simulink model "LHP_DT_v1"  (R2025b)
settings: Solver=VariableStepAuto  StartTime=0.0  StopTime=60  RelTol=1e-3
undefined symbols (not defined in the file): P
libraries: SignalEditorBlockLib x1
settings Model: Creator=RayAlmighty  LastModifiedBy=rayom

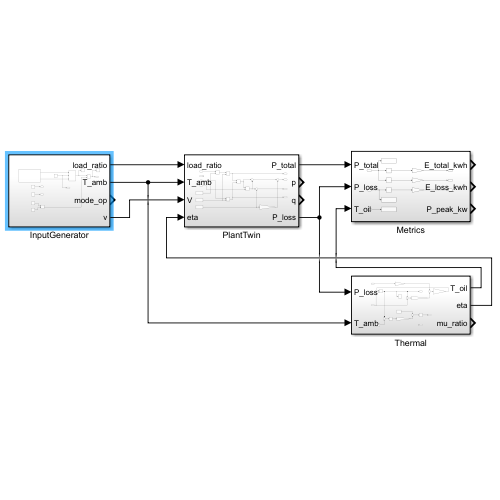
[thumbnail: Simulink's stored preview of the top-level diagram]
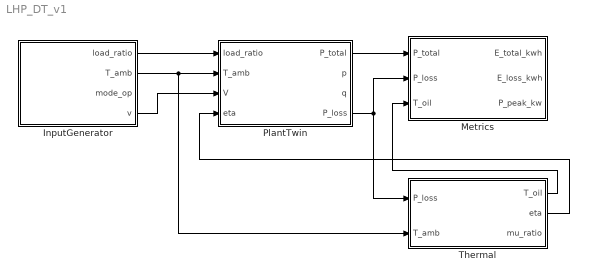
== system LHP_DT_v1 ==
  InputGenerator : Subsystem
  Metrics : Subsystem
  PlantTwin : Subsystem
  Thermal : Subsystem
  wires:
  InputGenerator/2(T_amb) -> Thermal/2(T_amb), PlantTwin/2(T_amb)
  InputGenerator/1(load_ratio) -> PlantTwin/1(load_ratio)
  InputGenerator/4(v) -> PlantTwin/3(V)
  Thermal/2(eta) -> PlantTwin/4(eta)
  PlantTwin/4(P_loss) -> Metrics/2(P_loss), Thermal/1(P_loss)
  PlantTwin/1(P_total) -> Metrics/1(P_total)
  Thermal/1(T_oil) -> Metrics/3(T_oil)

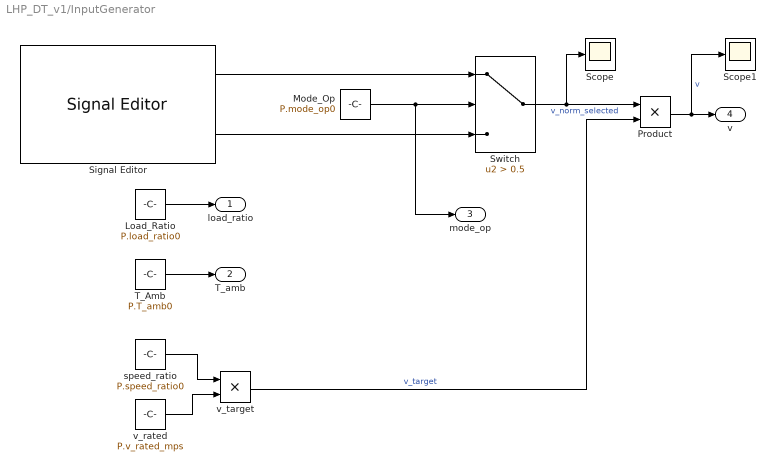
== system LHP_DT_v1/InputGenerator ==
  Load_Ratio : Constant  Value=P.load_ratio0
  Mode_Op : Constant  Value=P.mode_op0
  Product : Product
  Scope : Scope
      settings: ActiveDisplayYMinimum=-1  ActiveDisplayYMaximum=1
  Scope1 : Scope
      settings: ActiveDisplayYMinimum=-1  ActiveDisplayYMaximum=1  DataLoggingVariableName=ScopeData2
  Signal Editor : SignalEditorBlockLib/Signal Editor  FileName=v_norm.mat  ActiveScenario=Scenario  ActiveSignal=v_smooth  IsBus=off  OutputBusObjectStr=Bus: BusObject  SampleTime=0  ZeroCross=off  OutputAfterFinalValue=Setting to zero  Unit=inherit  PreserveSignalName=on  ApplySigPropsToAllScenarios=on  ApplySigPropsToAllSignals=off  SignalPropertySource=Dialog parameters
  Switch : Switch  Criteria=u2 > Threshold  Threshold=0.5  SaturateOnIntegerOverflow=off  InputSameDT=off
  T_Amb : Constant  Value=P.T_amb0
  speed_ratio : Constant  Value=P.speed_ratio0
  v_rated : Constant  Value=P.v_rated_mps
  v_target : Product
  load_ratio : Outport
  T_amb : Outport  Port=2
  mode_op : Outport  Port=3
  v : Outport  Port=4
  wires:
  Signal Editor/2 -> Switch/3
  Mode_Op/1 -> mode_op/1, Switch/2
  Switch/1 -> Product/1, Scope/1  "v_norm_selected"
  Load_Ratio/1 -> load_ratio/1
  T_Amb/1 -> T_amb/1
  speed_ratio/1 -> v_target/1
  v_rated/1 -> v_target/2
  v_target/1 -> Product/2  "v_target"
  Product/1 -> Scope1/1, v/1  "v"
  Signal Editor/1 -> Switch/1

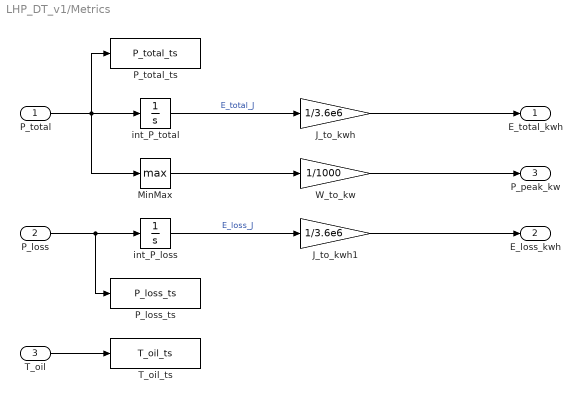
== system LHP_DT_v1/Metrics ==
  P_total : Inport
  P_loss : Inport  Port=2
  T_oil : Inport  Port=3
  J_to_kwh : Gain  Gain=1/3.6e6
  J_to_kwh1 : Gain  Gain=1/3.6e6
  MinMax : MinMax  Function=max
  P_loss_ts : ToWorkspace  VariableName=P_loss_ts  SaveFormat=Timeseries  SampleTime=-1
  P_total_ts : ToWorkspace  VariableName=P_total_ts  SaveFormat=Timeseries  SampleTime=-1
  T_oil_ts : ToWorkspace  VariableName=T_oil_ts  SaveFormat=Timeseries  SampleTime=-1
  W_to_kw : Gain  Gain=1/1000
  int_P_loss : Integrator
  int_P_total : Integrator
  E_total_kwh : Outport
  E_loss_kwh : Outport  Port=2
  P_peak_kw : Outport  Port=3
  wires:
  P_total/1 -> P_total_ts/1, int_P_total/1, MinMax/1
  int_P_total/1 -> J_to_kwh/1  "E_total_J"
  J_to_kwh/1 -> E_total_kwh/1
  P_loss/1 -> P_loss_ts/1, int_P_loss/1
  int_P_loss/1 -> J_to_kwh1/1  "E_loss_J"
  J_to_kwh1/1 -> E_loss_kwh/1
  MinMax/1 -> W_to_kw/1
  W_to_kw/1 -> P_peak_kw/1
  T_oil/1 -> T_oil_ts/1

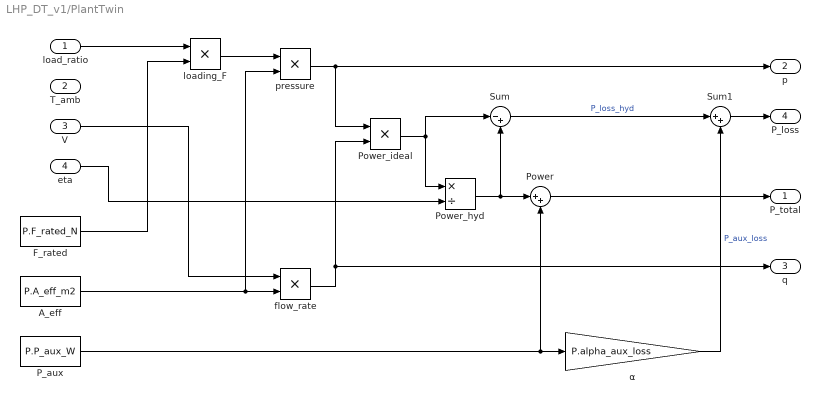
== system LHP_DT_v1/PlantTwin ==
  load_ratio : Inport
  T_amb : Inport  Port=2
  V : Inport  Port=3
  eta : Inport  Port=4
  A_eff : Constant  Value=P.A_eff_m2
  F_rated : Constant  Value=P.F_rated_N
  P_aux : Constant  Value=P.P_aux_W
  Power : Sum  Inputs=|++
  Power_hyd : Product  Inputs=*/
  Power_ideal : Product
  Sum : Sum  Inputs=|-+
  Sum1 : Sum  Inputs=|++
  flow_rate : Product
  loading_F : Product
  pressure : Product
  α : Gain  Gain=P.alpha_aux_loss
  P_total : Outport
  p : Outport  Port=2
  q : Outport  Port=3
  P_loss : Outport  Port=4
  wires:
  load_ratio/1 -> loading_F/1
  F_rated/1 -> loading_F/2
  loading_F/1 -> pressure/1
  A_eff/1 -> pressure/2, flow_rate/2
  V/1 -> flow_rate/1
  pressure/1 -> Power_ideal/1, p/1
  flow_rate/1 -> Power_ideal/2, q/1
  Power_ideal/1 -> Sum/1, Power_hyd/1
  P_aux/1 -> Power/2, α/1
  Power/1 -> P_total/1
  eta/1 -> Power_hyd/2
  Power_hyd/1 -> Sum/2, Power/1
  α/1 -> Sum1/2  "P_aux_loss"
  Sum/1 -> Sum1/1  "P_loss_hyd"
  Sum1/1 -> P_loss/1

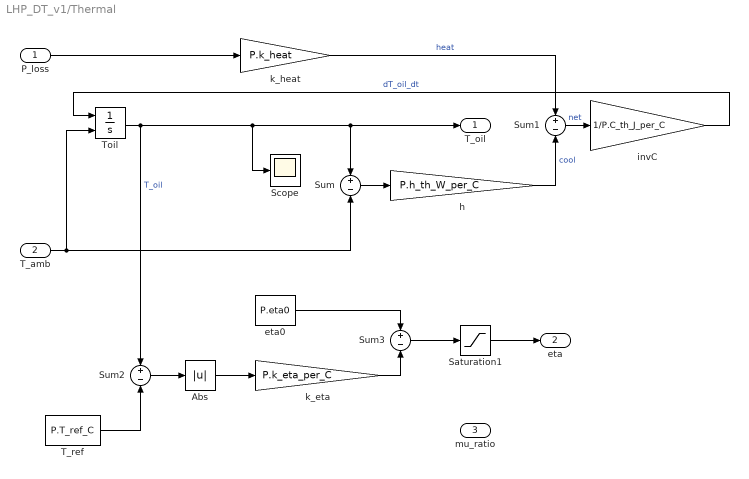
== system LHP_DT_v1/Thermal ==
  P_loss : Inport
  T_amb : Inport  Port=2
  Abs : Abs  SaturateOnIntegerOverflow=off
  Saturation1 : Saturate  UpperLimit=P.eta_max  LowerLimit=P.eta_min
  Scope : Scope
      settings: ActiveDisplayYMinimum=-1  ActiveDisplayYMaximum=1
  Sum{,1..3} (4 alike) : Sum  Inputs=+-
  T_ref : Constant  Value=P.T_ref_C
  Toil : Integrator  InitialConditionSource=external  InitialCondition=25
  eta0 : Constant  Value=P.eta0
  h : Gain  Gain=P.h_th_W_per_C
  invC : Gain  Gain=1/P.C_th_J_per_C
  k_eta : Gain  Gain=P.k_eta_per_C
  k_heat : Gain  Gain=P.k_heat
  T_oil : Outport
  eta : Outport  Port=2
  mu_ratio : Outport  Port=3
  wires:
  Toil/1 -> Scope/1, T_oil/1, Sum/1, Sum2/1  "T_oil"
  T_amb/1 -> Sum/2, Toil/2
  Sum/1 -> h/1
  k_heat/1 -> Sum1/1  "heat"
  h/1 -> Sum1/2  "cool"
  Sum1/1 -> invC/1  "net"
  invC/1 -> Toil/1  "dT_oil_dt"
  P_loss/1 -> k_heat/1
  T_ref/1 -> Sum2/2
  Sum2/1 -> Abs/1
  Abs/1 -> k_eta/1
  k_eta/1 -> Sum3/2
  eta0/1 -> Sum3/1
  Sum3/1 -> Saturation1/1
  Saturation1/1 -> eta/1
